simulink model "Rudder_system_control2020_3"  (R2020a)
settings: Solver=VariableStepAuto  StartTime=0.0  StopTime=300  MaxStep=0.02  RelTol=1e-3  AbsTol=1e-3  EnableMultiTasking=on
undefined symbols (not defined in the file or in its folder): Fg, H, Js, sigbuilder_block
libraries: fl_lib x76, nesl_utility x15, sh_lib x2
CloseFcn:
  | try,close(h1_ssc_hydraulic_actuator_analog_control),end
  | clear h1_ssc_hydraulic_actuator_analog_control
  | 
  | clear simlog_ssc_hydraulic_actuator_analog_control
Description:
  | Hydraulic Actuator with Analog Position Controller
settings Model: Creator=MathWorks  LastModifiedBy=victo
settings SolverCC: AutoScaleAbsTol=off  AlgebraicLoopSolver=LineSearch
settings DataIOCC: LimitDataPoints=on  SaveFormat=Array  ReturnWorkspaceOutputs=off
settings OptimizationCC: LifeSpan=inf
settings DebuggingCC: SolverPrmCheckMsg=warning  AllowSymbolicDim=off  PregeneratedLibrarySubsystemCodeDiagnostic=none  SFUnexpectedBacktrackingDiag=warning  SFNoUnconditionalDefaultTransitionDiag=warning  SFExecutionAtInitializationDiag=none  ArithmeticOperatorsInVariantConditions=warning
settings HardwareCC: ProdBitPerPointer=32  ProdBitPerSizeT=32  ProdBitPerPtrDiffT=32  ProdLargestAtomicFloat=None  ProdIntDivRoundTo=Undefined  ProdEndianess=Unspecified  ProdWordSize=32  ProdHWDeviceType=32-bit Generic
settings ModelReferenceCC: PropagateSignalLabelsOutOfModel=off
settings SFSimCC: SimUseLocalCustomCode=off  CustomCodeUndefinedFunction=UseInterfaceOnly
settings RTWCC: RTWUseLocalCustomCode=off
settings CodeAppCC: StateflowObjectComments=on
settings GRTTargetCC: TargetLangStandard=C89/C90 (ANSI)
settings ConfigComp: CovMetricSettings=dw  CovHtmlReporting=on  CovSaveCumulativeToWorkspaceVar=on  CovSaveSingleToWorkspaceVar=on  CovExternalEMLEnable=off  CovSFcnEnable=off
settings SimscapeCC: SimscapeLogType=all  SimscapeLogSimulationStatistics=on  SimscapeLogName=simlog_ssc_hydraulic_actuator_analog_control  SimscapeLogDataHistory=10000

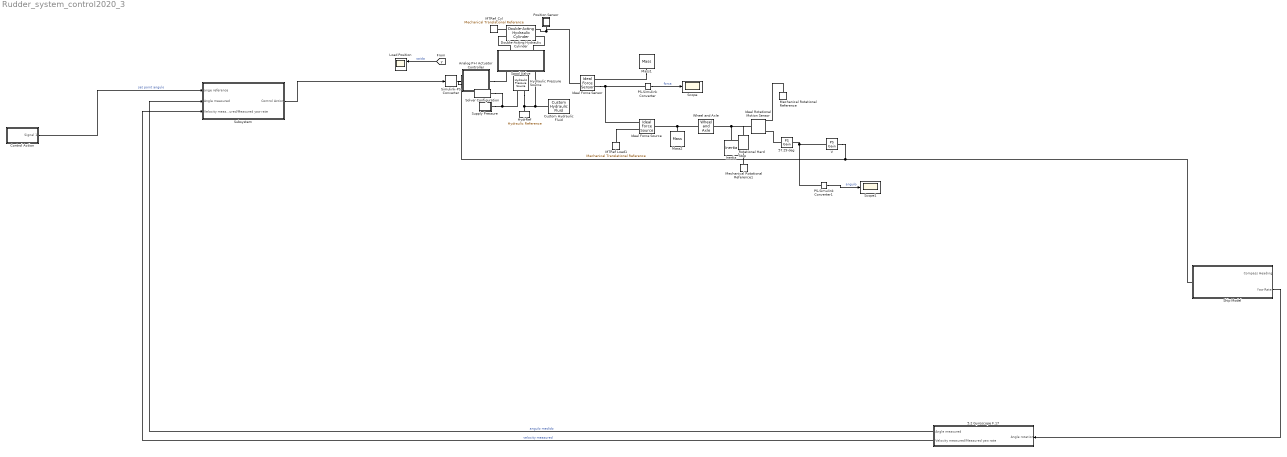
== system Rudder_system_control2020_3 ==
  5.2 Gyroscope F.17 : Subsystem
  57.29 deg : fl_lib/Physical Signals/Functions/PS Gain  gain=57.29 deg
      settings: SourceProductName=Foundation Library
  Analog P+I Actuator Controller : Subsystem
  Control Action : Subsystem  Tag=STV Subsys  LoadFcn=sigbuilder_block('load',[437.6 153 550.4 359.25 ]);  StartFcn=sigbuilder_block('start');  StopFcn=sigbuilder_block('stop');  ClipboardFcn=sigbuilder_block('clipboard');  mask(Sigbuilder block){tuvar=[0:10]}
      mask help: Simulink:masks:SigbuilderBlock_MD
      mask init:
      | if ~strcmp(get_param(bdroot(gcbh),'SimulationStatus'),'stopped') tuvar = sigbuilder_block('maskInit'); end
      settings: CopyFcn=sigbuilder_block('copy');  DeleteFcn=sigbuilder_block('delete');  ModelCloseFcn=sigbuilder_block('modelClose');  PreSaveFcn=sigbuilder_block('preSave');  PauseFcn=sigbuilder_block('pause');  ContinueFcn=sigbuilder_block('continue');  NameChangeFcn=sigbuilder_block('namechange');  OpenFcn=sigbuilder_block('open',[437.6 153 550.4 359.25 ]);  CloseFcn=sigbuilder_block('close');
      mask Display: plot(0, 0, 100, 100,[2, 2, 32, 32, 2], [68, 8, 8, 68, 68],[32, 2], [38, 38], [32, 19, 2],[53, 60, 44], [32, 17, 17, 2],[16, 16, 31, 31]);txt = getActiveGroup(gcbh);text(2, 100, txt,'verticalAlignment', 'top');
  Custom Hydraulic Fluid : fl_lib/Hydraulic/Hydraulic Utilities/Custom Hydraulic Fluid  density=850 kg/m^3  viscosity_kin=1.8e-05 m^2/s  bulk=8e+08 Pa  alpha=0.005  range_error=2
      settings: SourceProductName=Foundation Library  InternalSimscapePortConfiguration="{\"Bottom\":[],\"Left\":[],\"Right\":[{\"id\":\"G\",\"label\":\"\",\"type\":\"foundation.hydraulic.hydraulic\"}],\"Top\":[]}"
  Double-Acting Hydraulic Cylinder : sh_lib/Hydraulic Cylinders/Double-Acting Hydraulic Cylinder  area_A=PistonArea m^2  area_B=PistonArea m^2  stroke=PistonStroke m  init_pos=0 m  dead_vol_A=1e-4 m^3  dead_vol_B=1e-4 m^3  init_pressure_A=0 Pa  init_pressure_B=0 Pa  k_sh=1.4  stiff=1e6 N/m  D=150 N/(m/s)  hardstop_model=1  transition=0.1 mm  or=1
      settings: SourceProductBaseCode=SH  InternalSimscapePortConfiguration="{\"Bottom\":[],\"Left\":[{\"id\":\"C\",\"label\":\"C\",\"type\":\"foundation.mechanical.translational.translational\"},{\"id\":\"A\",\"label\":\"A\",\"type\":\"foundation.hydraulic.hydraulic\"}],\"Right\":[{\"id\":\"R\",\"label\":\"R\",\"type\":\"foundation.mechanical.translational.translational\"},{\"id\":\"B\",\"label\":\"B\",\"type\":\"foundation.hydraulic.hydraulic\"}],\"Top\":[]}"
  HydrRef : fl_lib/Hydraulic/Hydraulic Elements/Hydraulic Reference
      settings: SourceProductName=Foundation Library
  Hydraulic Pressure Source : fl_lib/Hydraulic/Hydraulic Sources/Hydraulic Pressure Source
      settings: SourceProductName=Foundation Library  InternalSimscapePortConfiguration="{\"Bottom\":[],\"Left\":[{\"id\":\"P\",\"label\":\"P\",\"type\":\"foundation.hydraulic.hydraulic\"}],\"Right\":[{\"id\":\"S\",\"label\":\"S\",\"type\":\"input\"},{\"id\":\"T\",\"label\":\"T\",\"type\":\"foundation.hydraulic.hydraulic\"}],\"Top\":[]}"
  Ideal Force Sensor : fl_lib/Mechanical/Mechanical Sensors/Ideal Force Sensor
  Ideal Force Source : fl_lib/Mechanical/Mechanical Sources/Ideal Force Source
  Ideal Rotational Motion Sensor : fl_lib/Mechanical/Mechanical Sensors/Ideal Rotational Motion Sensor  wrap_angle=simscape.enum.onoff.off  offset=0 rad
  Inertia : fl_lib/Mechanical/Rotational Elements/Inertia  inertia=Izz kg*m^2  w_specify=off  w_priority=High  w=0 rad/s  w_nominal_specify=off  w_nominal_unit=rad/s  w_nominal_value=1  t_specify=off  t_priority=None  t=0 N*m  t_nominal_specify=off  t_nominal_unit=N*m  t_nominal_value=1
  Load Position : Scope  NumInputPorts=2
  MTRef Load1 : fl_lib/Mechanical/Translational Elements/Mechanical Translational Reference
      settings: SourceProductName=Foundation Library
  MTRef_Cyl : fl_lib/Mechanical/Translational Elements/Mechanical Translational Reference
      settings: SourceProductName=Foundation Library
  Mass1 : fl_lib/Mechanical/Translational Elements/Mass  mass=PistonMass kg  v_specify=off  v_priority=High  v=0 m/s  v_nominal_specify=off  v_nominal_unit=m/s  v_nominal_value=1  f_specify=off  f_priority=High  f=0 N  f_nominal_specify=off  f_nominal_unit=N  f_nominal_value=1
      settings: SourceProductName=Foundation Library
  Mass2 : fl_lib/Mechanical/Translational Elements/Mass  mass=mrudder kg  v_specify=off  v_priority=High  v=0 m/s  v_nominal_specify=off  v_nominal_unit=m/s  v_nominal_value=1  f_specify=off  f_priority=High  f=0 N  f_nominal_specify=off  f_nominal_unit=N  f_nominal_value=1
      settings: SourceProductName=Foundation Library
  Mechanical Rotational Reference : fl_lib/Mechanical/Rotational Elements/Mechanical Rotational Reference
  Mechanical Rotational Reference1 : fl_lib/Mechanical/Rotational Elements/Mechanical Rotational Reference
  PS-Simulink Converter : nesl_utility/PS-Simulink Converter  PhysicalDomain=network_engine_domain  SubClassName=ps_output  LeftPortType=input  RightPortType=output  PseudoPeriodic=off  Frequencies=[]  Unit=inherit  AffineConversion=off
  PS-Simulink Converter1 : nesl_utility/PS-Simulink Converter  PhysicalDomain=network_engine_domain  SubClassName=ps_output  LeftPortType=input  RightPortType=output  PseudoPeriodic=off  Frequencies=[]  Unit=inherit  AffineConversion=off
  Position Sensor : Subsystem
      mask Display: disp('y')
  Rotational Hard Stop : fl_lib/Mechanical/Rotational Elements/Rotational Hard Stop  upper_bnd=30 deg  lower_bnd=-30 deg  stiff_up=1e6 N*m/rad  stiff_low=1e6 N*m/rad  D_up=0.01 N*m/(rad/s)  D_low=0.01 N*m/(rad/s)  model=simscape.enum.hardstop.smooth  transition=0.001 rad  w_specify=off  w_priority=None  w=0 rad/s  w_nominal_specify=off  w_nominal_unit=rad/s  w_nominal_value=1  t_specify=off  t_priority=None  t=0 N*m  t_nominal_specify=off  t_nominal_unit=N*m  t_nominal_value=1  phi_specify=off  phi_priority=High  phi=0 rad  phi_nominal_specify=off  phi_nominal_unit=rad  phi_nominal_value=1
      settings: SourceProductBaseCode=SS
  Scope : Scope
  Scope1 : Scope
  Ship Model : Subsystem
  Simulink-PS Converter : nesl_utility/Simulink-PS Converter  PhysicalDomain=network_engine_domain  SubClassName=ps_input  LeftPortType=input  RightPortType=output  PseudoPeriodic=off  Frequencies=[]  NoiseDistribution=none  NoiseParameters=[]  Unit=V  AffineConversion=off  FilteringAndDerivatives=zero  SimscapeFilterOrder=1  InputFilterTimeConstant=.001  UdotUserProvided=0
      settings: SourceProductName=Utilities
  Solver Configuration : nesl_utility/Solver Configuration  PhysicalDomain=network_engine_domain  SubClassName=solver  LeftPortType=input  RightPortType=generic  Tones=[]  Harmonics=[]  SimulateNoise=off  Profile=off  UseLocalSampling=off  EnableSwitchedLinearOptims=on  FrequencyDomain=off  UseCCode=off  RelTol=0.001  AbsTol=1e-06  MinStep=1e-09  ToWorkspace=off  RevertToSquareIcSolve=off  NumHomotopyIterations=100  PhasorMode=off  PhasorModeNumHarmonics=1  DoDC=off  ResidualTolerance=1e-9  UseLocalSolver=off  LocalSolverChoice=NE_BACKWARD_EULER_ADVANCER  LocalSolverSampleTime=0.001  DoFixedCost=off  MaxNonlinIter=3  MaxModeIter=2  LinearAlgebra=auto  EquationFormulation=NE_TIME_EF  DelaysMemoryBudget=1024  AutomaticFiltering=on  FilteringTimeConstant=0.001  PartitionStorageMethod=AS_NEEDED  PartitionMemoryBudget=1024  PartitionMethod=ROBUST
      settings: SourceProductName=Utilities
  Spool Valve : Subsystem  Tag=PublishSubsystem  mask(Single-Stage Servo Valve){K_V=0.5, x_max=0.5, A_max=9, x_lap=0.02, A_leak=0.25, G=0.5e-3/(pi/2), J=1e-4, lambda=0.01, R=10, L=2.5, Kt=0.04, R_controller=[10e3 10e3 10e3 100e3 50 100e3 10e3]}
      mask prompts: K_V "Flow Coefficient:"; x_max "Spool displacement limit (mm)"; A_max "Maximum orifice area (mm^2)"; x_lap "Spool displacement range for leakage (mm)"; A_leak "Leakage area at x=0 (mm^2)"; G "Spool displacement per motor rotation (m/radian)"; J "Total inertia reflected to motor (kg m^2)"; lambda "Total damping reflected to motor (Nm/(rad/s))"; R "Torque motor winding resistance (ohms)"; L "Torque motor winding inductance (H)"; Kt "Torque motor torque constant (Nm/A)"; R_controller "Motor controller resistance values [R1 R2 R3 R4 R5 R6 R7] (ohms)"
      mask help: Models a spool valve actuated directly by a torque motor.
      mask Display:
      | % Plot icon
      | plot([0;337.311462499201;337.311462499201;0;0], [566.910021007061;566.910021007061;0;0;566.910021007061])
      | plot([84.6585631370544;241.503668949008], [353;353])
      | plot([84.6585631370544;241.503668949008], [214;214])
      | plot([84.6585631370544;241.503668949008;241.503668949008;84.6585631370544;84.6585631370544], [491;491;76;76;491])
      | plot([84.6585631370544;241.503668949008], [449;449])
      | plot([241.503668949008;210.071657784283], [310;310])
      | plot([210.071657784283;210.071657784283;210.071657784283], [326;295;310.414731502533])
      | plot([241.503668949008;210.071657784283], [257;257])
      | plot([210.071657784283;210.071657784283;210.071657784283], [272;241;236.464468762279])
      | plot([84.6585631370544;115.964594297111], [257;257])
      | plot([115.964594297111;115.964594297111;115.964594297111], [272;241;236.464468762279])
      | plot([84.6585631370544;115.964594297111], [310;310])
      | plot([115.964594297111;115.964594297111;115.964594297111], [326;295;310.414731502533])
      | plot([84.6585631370544;241.503668949008], [185;110])
      | plot([241.503668949008;84.6585631370544], [185;110])
      | plot([84.6585631370544;241.503668949008], [395;395])
      | patch([85.0365031510592;110.547454096377;121.885654516518;85.0365031510592], [110;140;120;110], [0;0;0])
      | plot([85.0365031510592;110.547454096377;121.885654516518;85.0365031510592], [110;140;120;110])
      | patch([240.936758928001;204.087607562542;215.425807982683;240.936758928001], [109;120;140;109], [0;0;0])
      | 
      | plot([240.936758928001;204.087607562542;215.425807982683;240.936758928001], [109;120;140;109])
      | patch([83.6507230997086;127.554754726589;127.554754726589;83.6507230997086], [394;405;384;394], [0;0;0])
      | plot([83.6507230997086;127.554754726589;127.554754726589;83.6507230997086], [394;405;384;394])
      | patch([245.283069089055;201.253057457507;201.253057457507;245.283069089055], [451;461;440;451], [0;0;0])
      | plot([245.283069089055;201.253057457507;201.253057457507;245.283069089055], [451;461;440;451])
      | 
      | % Port labels
      | color('red')
      | port_label('LConn', 1,'S')
      | port_label('LConn', 2,'P')
      | port_label('LConn', 3,'T')
      | port_label('RConn', 1,'A')
      | port_label('RConn', 2,'B')
      | color('black')
  Subsystem : Subsystem
  Supply Pressure : Subsystem
  V : fl_lib/Physical Signals/Functions/PS Gain  gain=1 V
      settings: SourceProductName=Foundation Library
  Wheel and Axle : fl_lib/Mechanical/Mechanisms/Wheel and Axle  R=0.05 m  or=1  t_specify=off  t_priority=None  t=0 N*m  t_nominal_specify=off  t_nominal_unit=N*m  t_nominal_value=1  f_specify=off  f_priority=None  f=0 N  f_nominal_specify=off  f_nominal_unit=N  f_nominal_value=1
  wires:
  [y] -> Load Position/1  "saida"
  PS-Simulink Converter/1 -> Scope/1  "forca"
  PS-Simulink Converter1/1 -> Scope1/1  "angulo"
  Subsystem/1(Control Action) -> Simulink-PS Converter/1
  5.2 Gyroscope F.17/1(Angle measured) -> Subsystem/2(Angle measured)  "angulo medido"
  5.2 Gyroscope F.17/2(Velocity measured/Measured yaw rate) -> Subsystem/3(Velocity measured/Measured yaw rate)  "velocity measured"
  Control Action/1(Signal 1) -> Subsystem/1(ange reference)  "set point angulo"
  Ship Model/2(Yaw Rate) -> 5.2 Gyroscope F.17/1(Angle rotation)
  connections:
  Custom Hydraulic Fluid/RConn1 -- Hydraulic Pressure Source/RConn2 -- HydrRef/LConn1 -- Spool Valve/LConn3
  Spool Valve/RConn2 -- Double-Acting Hydraulic Cylinder/RConn2
  Spool Valve/RConn1 -- Double-Acting Hydraulic Cylinder/LConn2
  Simulink-PS Converter/RConn1 -- Analog P+I Actuator Controller/LConn2
  Hydraulic Pressure Source/LConn1 -- Spool Valve/LConn2
  Position Sensor/RConn1 -- Ideal Force Sensor/LConn1 -- Double-Acting Hydraulic Cylinder/RConn1
  Supply Pressure/RConn1 -- Solver Configuration/RConn1 -- Hydraulic Pressure Source/RConn1
  Double-Acting Hydraulic Cylinder/LConn1 -- MTRef_Cyl/LConn1
  Ideal Force Sensor/RConn2 -- Ideal Force Source/RConn1 -- PS-Simulink Converter/LConn1
  Mass1/LConn1 -- Ideal Force Sensor/RConn1
  MTRef Load1/LConn1 -- Ideal Force Source/RConn2
  Mass2/LConn1 -- Wheel and Axle/RConn1 -- Ideal Force Source/LConn1
  Inertia/LConn1 -- Rotational Hard Stop/LConn1 -- Ideal Rotational Motion Sensor/LConn1 -- Wheel and Axle/LConn1
  Mechanical Rotational Reference/LConn1 -- Ideal Rotational Motion Sensor/RConn1
  57.29 deg/LConn1 -- Ideal Rotational Motion Sensor/RConn3
  PS-Simulink Converter1/LConn1 -- V/LConn1 -- 57.29 deg/RConn1
  Mechanical Rotational Reference1/LConn1 -- Rotational Hard Stop/RConn1
  V/RConn1 -- Ship Model/LConn1 -- Analog P+I Actuator Controller/LConn1
  Analog P+I Actuator Controller/RConn1 -- Spool Valve/LConn1

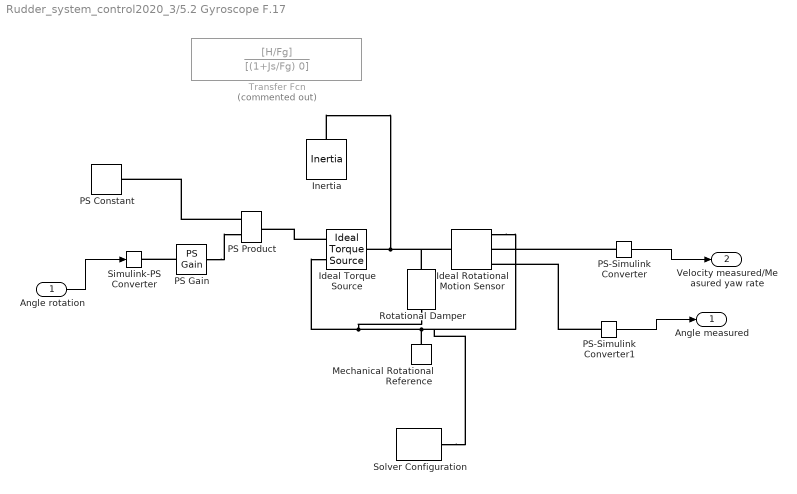
== system Rudder_system_control2020_3/5.2 Gyroscope F.17 ==
  Angle rotation : Inport
  Ideal Rotational Motion Sensor : fl_lib/Mechanical/Mechanical Sensors/Ideal Rotational Motion Sensor  wrap_angle=simscape.enum.onoff.off  offset=0 rad
  Ideal Torque Source : fl_lib/Mechanical/Mechanical Sources/Ideal Torque Source
  Inertia : fl_lib/Mechanical/Rotational Elements/Inertia  inertia=0.08 kg*m^2  w_specify=off  w_priority=High  w=0 rad/s  w_nominal_specify=off  w_nominal_unit=rad/s  w_nominal_value=1  t_specify=off  t_priority=None  t=0 N*m  t_nominal_specify=off  t_nominal_unit=N*m  t_nominal_value=1
  Mechanical Rotational Reference : fl_lib/Mechanical/Rotational Elements/Mechanical Rotational Reference
  PS Constant : fl_lib/Physical Signals/Sources/PS Constant  constant=1
  PS Gain : fl_lib/Physical Signals/Functions/PS Gain  gain=0.017
  PS Product : fl_lib/Physical Signals/Functions/PS Product
  PS-Simulink Converter : nesl_utility/PS-Simulink Converter  PhysicalDomain=network_engine_domain  SubClassName=ps_output  LeftPortType=input  RightPortType=output  PseudoPeriodic=off  Frequencies=[]  Unit=inherit  AffineConversion=off
  PS-Simulink Converter1 : nesl_utility/PS-Simulink Converter  PhysicalDomain=network_engine_domain  SubClassName=ps_output  LeftPortType=input  RightPortType=output  PseudoPeriodic=off  Frequencies=[]  Unit=inherit  AffineConversion=off
  Rotational Damper : fl_lib/Mechanical/Rotational Elements/Rotational Damper  D=1 N*m/(rad/s)  w_specify=off  w_priority=None  w=0 rad/s  w_nominal_specify=off  w_nominal_unit=rad/s  w_nominal_value=1  t_specify=off  t_priority=None  t=0 N*m  t_nominal_specify=off  t_nominal_unit=N*m  t_nominal_value=1
  Simulink-PS Converter : nesl_utility/Simulink-PS Converter  PhysicalDomain=network_engine_domain  SubClassName=ps_input  LeftPortType=input  RightPortType=output  PseudoPeriodic=off  Frequencies=[]  NoiseDistribution=none  NoiseParameters=[]  Unit=1  AffineConversion=off  FilteringAndDerivatives=provide  SimscapeFilterOrder=1  InputFilterTimeConstant=0.001  UdotUserProvided=0
  Solver Configuration : nesl_utility/Solver Configuration  PhysicalDomain=network_engine_domain  SubClassName=solver  LeftPortType=input  RightPortType=generic  Tones=[]  Harmonics=[]  SimulateNoise=off  Profile=off  UseLocalSampling=off  EnableSwitchedLinearOptims=on  FrequencyDomain=off  UseCCode=off  RelTol=0.001  AbsTol=1e-06  MinStep=1e-09  ToWorkspace=off  RevertToSquareIcSolve=off  NumHomotopyIterations=100  PhasorMode=off  PhasorModeNumHarmonics=1  DoDC=off  ResidualTolerance=1e-09  UseLocalSolver=off  LocalSolverChoice=NE_BACKWARD_EULER_ADVANCER  LocalSolverSampleTime=0.001  DoFixedCost=off  MaxNonlinIter=3  MaxModeIter=2  LinearAlgebra=auto  EquationFormulation=NE_TIME_EF  DelaysMemoryBudget=1024  AutomaticFiltering=on  FilteringTimeConstant=0.001  PartitionStorageMethod=AS_NEEDED  PartitionMemoryBudget=1024  PartitionMethod=ROBUST
  Transfer Fcn : TransferFcn  Commented=on  Numerator=[H/Fg]  Denominator=[(1+Js/Fg) 0]
  Angle measured : Outport
  Velocity measured/Measured yaw rate : Outport  Port=2
  wires:
  Angle rotation/1 -> Simulink-PS Converter/1
  PS-Simulink Converter/1 -> Velocity measured/Measured yaw rate/1
  PS-Simulink Converter1/1 -> Angle measured/1
  connections:
  PS Product/LConn1 -- PS Constant/RConn1
  PS Gain/LConn1 -- Simulink-PS Converter/RConn1
  PS Gain/RConn1 -- PS Product/LConn2
  Ideal Torque Source/RConn1 -- PS Product/RConn1
  Mechanical Rotational Reference/LConn1 -- Solver Configuration/RConn1 -- Ideal Rotational Motion Sensor/RConn1 -- Rotational Damper/RConn1 -- Ideal Torque Source/RConn2
  Inertia/LConn1 -- Rotational Damper/LConn1 -- Ideal Rotational Motion Sensor/LConn1 -- Ideal Torque Source/LConn1
  PS-Simulink Converter/LConn1 -- Ideal Rotational Motion Sensor/RConn2
  PS-Simulink Converter1/LConn1 -- Ideal Rotational Motion Sensor/RConn3

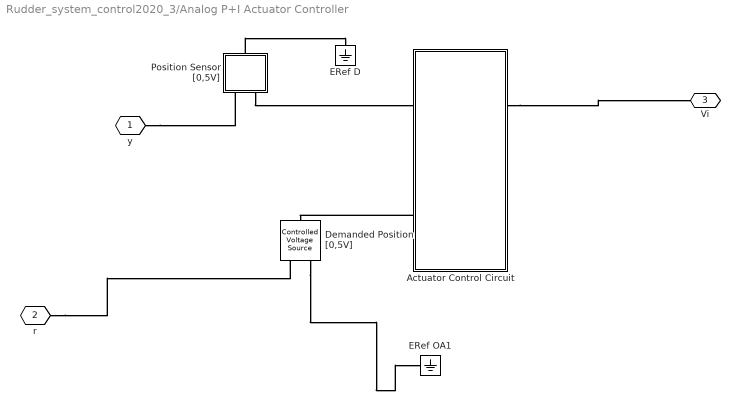
== system Rudder_system_control2020_3/Analog P+I Actuator Controller ==
  Actuator Control Circuit : Subsystem  Tag=PublishSubsystem
  Demanded Position [0,5V] : fl_lib/Electrical/Electrical Sources/Controlled Voltage Source
      settings: SourceProductName=Foundation Library
  ERef D : fl_lib/Electrical/Electrical Elements/Electrical Reference
      settings: SourceProductName=Foundation Library
  ERef OA1 : fl_lib/Electrical/Electrical Elements/Electrical Reference
      settings: SourceProductName=Foundation Library
  Position Sensor [0,5V] : Subsystem
  y : PMIOPort  Tag=PMCPort  Side=Left
  r : PMIOPort  Tag=PMCPort  Port=2  Side=Left
  Vi : PMIOPort  Port=3  Side=Right
  connections:
  y/RConn1 -- Position Sensor [0,5V]/LConn1
  r/RConn1 -- Demanded Position [0,5V]/RConn1
  Actuator Control Circuit/LConn2 -- Demanded Position [0,5V]/LConn1
  Position Sensor [0,5V]/RConn1 -- ERef D/LConn1
  Position Sensor [0,5V]/LConn2 -- Actuator Control Circuit/LConn1
  Actuator Control Circuit/RConn1 -- Vi/RConn1
  Demanded Position [0,5V]/RConn2 -- ERef OA1/LConn1

== system Rudder_system_control2020_3/Control Action ==
  Demux : Demux  Tag=STV Demux  Outputs=1
      settings: DisplayOption=none
  FromWs : FromWorkspace  Tag=STV FromWs  VariableName=tuvar
      SigBuilderData=|
      | common.afterFinalStr = 'Extrapolate'
      | common.sampleTime = 0
      | dataSet.timeRange = [0 10]
      | dataSet.name = 'Group 1'
      | sbobj.Groups.Name = 'Group 1'
      | sbobj.Groups.Signals.Name = 'Signal 1'
      | sbobj.Groups.Signals.XData = [0 1.02 1.02 10]
      | sbobj.Groups.Signals.YData = [0 0 1 1]
  Signal 1 : Outport  Tag=STV Outport
  wires:
  Demux/1 -> Signal 1/1
  FromWs/1 -> Demux/1

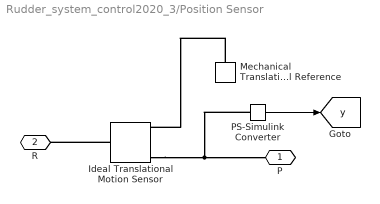
== system Rudder_system_control2020_3/Position Sensor ==
  Ideal Translational Motion Sensor : fl_lib/Mechanical/Mechanical Sensors/Ideal Translational Motion Sensor  offset=0 m
  Mechanical Translational Reference : fl_lib/Mechanical/Translational Elements/Mechanical Translational Reference
  PS-Simulink Converter : nesl_utility/PS-Simulink Converter  PhysicalDomain=network_engine_domain  SubClassName=ps_output  LeftPortType=input  RightPortType=output  PseudoPeriodic=off  Frequencies=[]  Unit=inherit  AffineConversion=off
  P : PMIOPort  Side=Left
  R : PMIOPort  Port=2  Side=Right
  tag scope: y=global
  wires:
  PS-Simulink Converter/1 -> [y]
  connections:
  Ideal Translational Motion Sensor/LConn1 -- R/RConn1
  Ideal Translational Motion Sensor/RConn3 -- PS-Simulink Converter/LConn1 -- P/RConn1
  Mechanical Translational Reference/LConn1 -- Ideal Translational Motion Sensor/RConn1

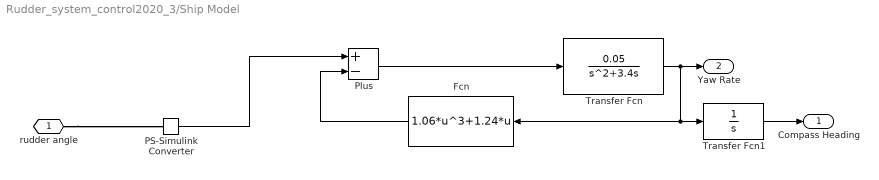
== system Rudder_system_control2020_3/Ship Model ==
  Fcn : Fcn  Expr=1.06*u^3+1.24*u
  PS-Simulink Converter : nesl_utility/PS-Simulink Converter  PhysicalDomain=network_engine_domain  SubClassName=ps_output  LeftPortType=input  RightPortType=output  PseudoPeriodic=off  Frequencies=[]  Unit=inherit  AffineConversion=off
  Plus : Sum  Inputs=+-
  Transfer Fcn : TransferFcn  Numerator=[0.05]  Denominator=[1 3.4 0]
  Transfer Fcn1 : TransferFcn  Denominator=[1 0]
  rudder angle : PMIOPort  Side=Left
  Compass Heading : Outport
  Yaw Rate : Outport  Port=2
  wires:
  Transfer Fcn1/1 -> Compass Heading/1
  Fcn/1 -> Plus/2
  Transfer Fcn/1 -> Fcn/1, Transfer Fcn1/1, Yaw Rate/1
  Plus/1 -> Transfer Fcn/1
  PS-Simulink Converter/1 -> Plus/1
  connections:
  rudder angle/RConn1 -- PS-Simulink Converter/LConn1

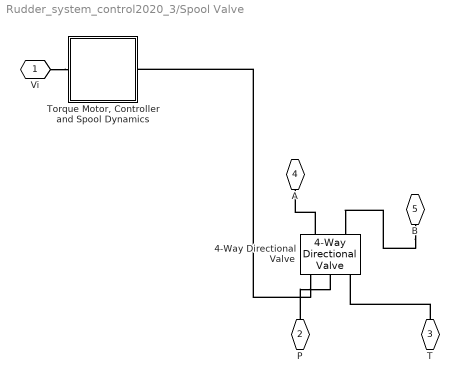
== system Rudder_system_control2020_3/Spool Valve ==
  4-Way Directional Valve : sh_lib/Valves/Directional Valves/4-Way Directional Valve  area_spec=sh.valves.directional_valves.enum.area_spec.identical  x_0_P_A=0 m  x_0_P_B=0 m  x_0_A_T=0 m  x_0_B_T=0 m  mdl_type_identical=sh.valves.directional_valves.enum.mdl_type.linear  mdl_type_different=sh.valves.directional_valves.enum.mdl_type.linear  opening_max=0.005 m  area_max=0.5e-4 m^2  opening_max_P_A=0.005 m  area_max_P_A=0.5e-4 m^2  opening_max_P_B=0.005 m  area_max_P_B=0.5e-4 m^2  opening_max_A_T=0.005 m  area_max_A_T=0.5e-4 m^2  opening_max_B_T=0.005 m  area_max_B_T=0.5e-4 m^2  opening_area_tab=[-.002, 0, .002, .005, .015] m  area_tab=[1e-09, 2.0352e-07, 4.0736e-05, .00011438, .00034356] m^2  opening_flow_rate_tab=[-.002, 0, .002, .005, .015] m  pressure_tab=[-10000000, -5000000, -2000000, 2000000, 5000000, 10000000] Pa  flow_rate_tab=[-1e-07, -7.0711e-08, -4.4721e-08, 4.4721e-08, 7.0711e-08, 1e-07; -2.0352e-05, -1.4391e-05, -9.1017e-06, 9.1017e-06, 1.4391e-05, 2.0352e-05; -.0040736, -.0028805, -.0018218, .0018218, .0028805, .0040736; -.011438, -.0080879, -.0051152, .0051152, .0080879, .011438; -.034356, -.024293, -.015364, .015364, .024293, .034356] m^3/s  opening_area_tab_P_A=[-.002, 0, .002, .005, .015] m  area_tab_P_A=[1e-09, 2.0352e-07, 4.0736e-05, .00011438, .00034356] m^2  opening_flow_rate_tab_P_A=[-.002, 0, .002, .005, .015] m  pressure_tab_P_A=[-10000000, -5000000, -2000000, 2000000, 5000000, 10000000] Pa  flow_rate_tab_P_A=[-1e-07, -7.0711e-08, -4.4721e-08, 4.4721e-08, 7.0711e-08, 1e-07; -2.0352e-05, -1.4391e-05, -9.1017e-06, 9.1017e-06, 1.4391e-05, 2.0352e-05; -.0040736, -.0028805, -.0018218, .0018218, .0028805, .0040736; -.011438, -.0080879, -.0051152, .0051152, .0080879, .011438; -.034356, -.024293, -.015364, .015364, .024293, .034356] m^3/s  opening_area_tab_P_B=[-.002, 0, .002, .005, .015] m  area_tab_P_B=[1e-09, 2.0352e-07, 4.0736e-05, .00011438, .00034356] m^2  opening_flow_rate_tab_P_B=[-.002, 0, .002, .005, .015] m  pressure_tab_P_B=[-10000000, -5000000, -2000000, 2000000, 5000000, 10000000] Pa  flow_rate_tab_P_B=[-1e-07, -7.0711e-08, -4.4721e-08, 4.4721e-08, 7.0711e-08, 1e-07; -2.0352e-05, -1.4391e-05, -9.1017e-06, 9.1017e-06, 1.4391e-05, 2.0352e-05; -.0040736, -.0028805, -.0018218, .0018218, .0028805, .0040736; -.011438, -.0080879, -.0051152, .0051152, .0080879, .011438; -.034356, -.024293, -.015364, .015364, .024293, .034356] m^3/s  opening_area_tab_A_T=[-.002, 0, .002, .005, .015] m  area_tab_A_T=[1e-09, 2.0352e-07, 4.0736e-05, .00011438, .00034356] m^2  opening_flow_rate_tab_A_T=[-.002, 0, .002, .005, .015] m  pressure_tab_A_T=[-10000000, -5000000, -2000000, 2000000, 5000000, 10000000] Pa  flow_rate_tab_A_T=[-1e-07, -7.0711e-08, -4.4721e-08, 4.4721e-08, 7.0711e-08, 1e-07; -2.0352e-05, -1.4391e-05, -9.1017e-06, 9.1017e-06, 1.4391e-05, 2.0352e-05; -.0040736, -.0028805, -.0018218, .0018218, .0028805, .0040736; -.011438, -.0080879, -.0051152, .0051152, .0080879, .011438; -.034356, -.024293, -.015364, .015364, .024293, .034356] m^3/s  opening_area_tab_B_T=[-.002, 0, .002, .005, .015] m  area_tab_B_T=[1e-09, 2.0352e-07, 4.0736e-05, .00011438, .00034356] m^2  opening_flow_rate_tab_B_T=[-.002, 0, .002, .005, .015] m  pressure_tab_B_T=[-10000000, -5000000, -2000000, 2000000, 5000000, 10000000] Pa  flow_rate_tab_B_T=[-1e-07, -7.0711e-08, -4.4721e-08, 4.4721e-08, 7.0711e-08, 1e-07; -2.0352e-05, -1.4391e-05, -9.1017e-06, 9.1017e-06, 1.4391e-05, 2.0352e-05; -.0040736, -.0028805, -.0018218, .0018218, .0028805, .0040736; -.011438, -.0080879, -.0051152, .0051152, .0080879, .011438; -.034356, -.024293, -.015364, .015364, .024293, .034356] m^3/s  interp_method_identical=sh.valves.directional_valves.enum.interp_method.linear  interp_method_different=sh.valves.directional_valves.enum.interp_method.linear  extrap_method_identical=sh.valves.directional_valves.enum.extrap_method.linear  extrap_method_different=sh.valves.directional_valves.enum.extrap_method.linear  A_leak=1e-12 m^2  C_d=0.7  lam_spec=sh.valves.directional_valves.enum.lam_spec.pressure_ratio  B_lam=0.999  Re_cr=12
      settings: SourceProductBaseCode=SH  InternalSimscapePortConfiguration="{\"Bottom\":[],\"Left\":[{\"id\":\"A\",\"label\":\"A\",\"type\":\"foundation.hydraulic.hydraulic\"},{\"id\":\"B\",\"label\":\"B\",\"type\":\"foundation.hydraulic.hydraulic\"}],\"Right\":[{\"id\":\"S\",\"label\":\"S\",\"type\":\"input\"},{\"id\":\"P\",\"label\":\"P\",\"type\":\"foundation.hydraulic.hydraulic\"},{\"id\":\"T\",\"label\":\"T\",\"type\":\"foundation.hydraulic.hydraulic\"}],\"Top\":[]}"
  "Torque Motor, Controller and Spool Dynamics" : Subsystem
  Vi : PMIOPort  Tag=PMCPort  Side=Left
  P : PMIOPort  Tag=PMCPort  Port=2  Side=Left
  T : PMIOPort  Tag=PMCPort  Port=3  Side=Left
  A : PMIOPort  Tag=PMCPort  Port=4  Side=Right
  B : PMIOPort  Tag=PMCPort  Port=5  Side=Right
  connections:
  Vi/RConn1 -- "Torque Motor, Controller and Spool Dynamics"/LConn1
  4-Way Directional Valve/RConn1 -- "Torque Motor, Controller and Spool Dynamics"/RConn1
  4-Way Directional Valve/LConn1 -- A/RConn1
  B/RConn1 -- 4-Way Directional Valve/LConn2
  P/RConn1 -- 4-Way Directional Valve/RConn2
  T/RConn1 -- 4-Way Directional Valve/RConn3

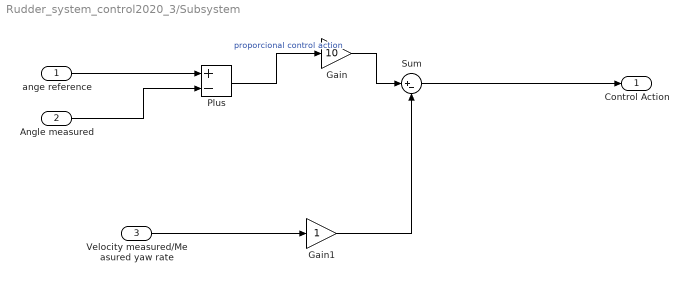
== system Rudder_system_control2020_3/Subsystem ==
  ange reference : Inport
  Angle measured : Inport  Port=2
  Velocity measured/Measured yaw rate : Inport  Port=3
  Gain : Gain  Gain=10
  Gain1 : Gain
  Plus : Sum  Inputs=+-
  Sum : Sum  Inputs=|+-
  Control Action : Outport
  wires:
  Sum/1 -> Control Action/1
  Plus/1 -> Gain/1  "proporcional control action"
  ange reference/1 -> Plus/1
  Angle measured/1 -> Plus/2
  Gain/1 -> Sum/1
  Gain1/1 -> Sum/2
  Velocity measured/Measured yaw rate/1 -> Gain1/1

== system Rudder_system_control2020_3/Supply Pressure ==
  Supply Pressure : Constant  Value=200
  bar : nesl_utility/Simulink-PS Converter  PhysicalDomain=network_engine_domain  SubClassName=ps_input  LeftPortType=input  RightPortType=output  PseudoPeriodic=off  Frequencies=[]  NoiseDistribution=none  NoiseParameters=[]  Unit=bar  AffineConversion=off  FilteringAndDerivatives=zero  SimscapeFilterOrder=1  InputFilterTimeConstant=.001  UdotUserProvided=0
      settings: SourceProductName=Utilities
  S : PMIOPort  Side=Right
  wires:
  Supply Pressure/1 -> bar/1
  connections:
  bar/RConn1 -- S/RConn1

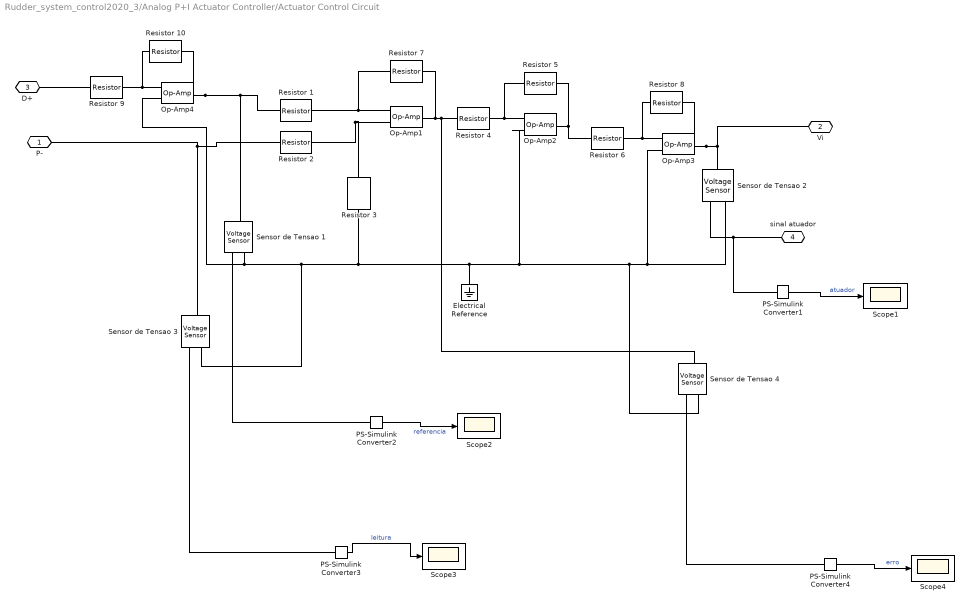
== system Rudder_system_control2020_3/Analog P+I Actuator Controller/Actuator Control Circuit ==
  Electrical Reference : fl_lib/Electrical/Electrical Elements/Electrical Reference
  Op-Amp{1..4} (4 alike) : fl_lib/Electrical/Electrical Elements/Op-Amp  outI_specify=off  outI_priority=None  outI=0 A  outI_nominal_specify=off  outI_nominal_unit=A  outI_nominal_value=1
  PS-Simulink Converter{1..4} (4 alike) : nesl_utility/PS-Simulink Converter  PhysicalDomain=network_engine_domain  SubClassName=ps_output  LeftPortType=input  RightPortType=output  PseudoPeriodic=off  Frequencies=[]  Unit=inherit  AffineConversion=off
  Resistor {1..10} (10 alike) : fl_lib/Electrical/Electrical Elements/Resistor  R=1 Ohm  i_specify=off  i_priority=None  i=0 A  i_nominal_specify=off  i_nominal_unit=A  i_nominal_value=1  v_specify=off  v_priority=None  v=0 V  v_nominal_specify=off  v_nominal_unit=V  v_nominal_value=1
  Scope{1..4} (4 alike) : Scope
  Sensor de Tensao {1..4} (4 alike) : fl_lib/Electrical/Electrical Sensors/Voltage Sensor
  P- : PMIOPort  Side=Left
  Vi : PMIOPort  Port=2  Side=Right
  D+ : PMIOPort  Port=3  Side=Left
  sinal atuador : PMIOPort  Port=4  Side=Right
  wires:
  PS-Simulink Converter1/1 -> Scope1/1  "atuador"
  PS-Simulink Converter2/1 -> Scope2/1  "referencia"
  PS-Simulink Converter3/1 -> Scope3/1  "leitura"
  PS-Simulink Converter4/1 -> Scope4/1  "erro"
  connections:
  D+/RConn1 -- Resistor 9/LConn1
  Resistor 9/RConn1 -- Resistor 10/LConn1 -- Op-Amp4/LConn2
  Resistor 5/RConn1 -- Op-Amp2/RConn1 -- Resistor 6/LConn1
  Resistor 6/RConn1 -- Resistor 8/LConn1 -- Op-Amp3/LConn2
  Op-Amp1/RConn1 -- Resistor 7/RConn1 -- Resistor 4/LConn1 -- Sensor de Tensao 4/LConn1
  Op-Amp3/RConn1 -- Resistor 8/RConn1 -- Vi/RConn1 -- Sensor de Tensao 2/LConn1
  Resistor 2/RConn1 -- Op-Amp1/LConn1 -- Resistor 3/LConn1
  Op-Amp4/LConn1 -- Sensor de Tensao 1/RConn2 -- Sensor de Tensao 3/RConn2 -- Resistor 3/RConn1 -- Electrical Reference/LConn1 -- Op-Amp2/LConn1 -- Sensor de Tensao 4/RConn2 -- Sensor de Tensao 2/RConn2 -- Op-Amp3/LConn1
  Resistor 5/LConn1 -- Op-Amp2/LConn2 -- Resistor 4/RConn1
  Op-Amp1/LConn2 -- Resistor 7/LConn1 -- Resistor 1/RConn1
  sinal atuador/RConn1 -- Sensor de Tensao 2/RConn1 -- PS-Simulink Converter1/LConn1
  Op-Amp4/RConn1 -- Resistor 10/RConn1 -- Sensor de Tensao 1/LConn1 -- Resistor 1/LConn1
  Resistor 2/LConn1 -- Sensor de Tensao 3/LConn1 -- P-/RConn1
  Sensor de Tensao 1/RConn1 -- PS-Simulink Converter2/LConn1
  Sensor de Tensao 3/RConn1 -- PS-Simulink Converter3/LConn1
  Sensor de Tensao 4/RConn1 -- PS-Simulink Converter4/LConn1

== system Rudder_system_control2020_3/Analog P+I Actuator Controller/Position Sensor [0,5V] ==
  Controlled Voltage Source : fl_lib/Electrical/Electrical Sources/Controlled Voltage Source
      settings: SourceProductName=Foundation Library
  + : PMIOPort  Side=Right
  y : PMIOPort  Port=2  Side=Left
  - : PMIOPort  Port=3  Side=Left
  connections:
  +/RConn1 -- Controlled Voltage Source/LConn1
  -/RConn1 -- Controlled Voltage Source/RConn2
  Controlled Voltage Source/RConn1 -- y/RConn1

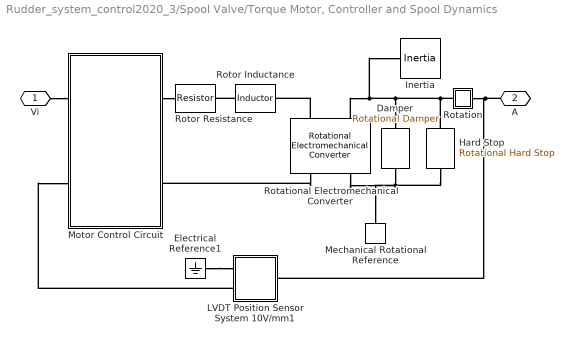
== system Rudder_system_control2020_3/Spool Valve/Torque Motor, Controller and Spool Dynamics ==
  Damper : fl_lib/Mechanical/Rotational Elements/Rotational Damper  D=lambda N*m/(rad/s)  w_specify=off  w_priority=High  w=0 rad/s  w_nominal_specify=off  w_nominal_unit=rad/s  w_nominal_value=1  t_specify=off  t_priority=High  t=0 N*m  t_nominal_specify=off  t_nominal_unit=N*m  t_nominal_value=1
      settings: SourceProductName=Foundation Library
  Electrical Reference1 : fl_lib/Electrical/Electrical Elements/Electrical Reference
      settings: SourceProductName=Foundation Library
  Hard Stop : fl_lib/Mechanical/Rotational Elements/Rotational Hard Stop  upper_bnd=x_max*1e-3/G rad  lower_bnd=-x_max*1e-3/G rad  stiff_up=1e+06 N*m/rad  stiff_low=1e+6 N*m/rad  D_up=0.05 N*m/(rad/s)  D_low=0.05 N*m/(rad/s)  model=3  transition=0.001 rad  w_specify=off  w_priority=High  w=0 rad/s  w_nominal_specify=off  w_nominal_unit=rad/s  w_nominal_value=1  t_specify=off  t_priority=High  t=0 N*m  t_nominal_specify=off  t_nominal_unit=N*m  t_nominal_value=1  phi_specify=on  phi_priority=High  phi=0 rad  phi_nominal_specify=off  phi_nominal_unit=rad  phi_nominal_value=1
      settings: SourceProductName=Foundation Library
  Inertia : fl_lib/Mechanical/Rotational Elements/Inertia  inertia=J kg*m^2  w_specify=off  w_priority=High  w=0 rad/s  w_nominal_specify=off  w_nominal_unit=rad/s  w_nominal_value=1  t_specify=off  t_priority=High  t=0 N*m  t_nominal_specify=off  t_nominal_unit=N*m  t_nominal_value=1
      settings: SourceProductName=Foundation Library
  LVDT Position Sensor System 10V/mm1 : Subsystem
  Mechanical Rotational Reference : fl_lib/Mechanical/Rotational Elements/Mechanical Rotational Reference
      settings: SourceProductName=Foundation Library
  Motor Control Circuit : Subsystem  Tag=PublishSubsystem
  Rotation : Subsystem
      mask Display: disp('A')
  Rotational Electromechanical Converter : fl_lib/Electrical/Electrical Elements/Rotational Electromechanical Converter  K=Kt V/(rad/s)  i_specify=off  i_priority=High  i=0 A  i_nominal_specify=off  i_nominal_unit=A  i_nominal_value=1  v_specify=off  v_priority=High  v=0 V  v_nominal_specify=off  v_nominal_unit=V  v_nominal_value=1  t_specify=off  t_priority=High  t=0 N*m  t_nominal_specify=off  t_nominal_unit=N*m  t_nominal_value=1  w_specify=off  w_priority=High  w=0 rad/s  w_nominal_specify=off  w_nominal_unit=rad/s  w_nominal_value=1
      settings: SourceProductName=Foundation Library
  Rotor Inductance : fl_lib/Electrical/Electrical Elements/Inductor  l=L H  r=0 Ohm  g=1e-09 1/Ohm  i_specify=off  i_priority=High  i=0 A  i_nominal_specify=off  i_nominal_unit=A  i_nominal_value=1  v_specify=off  v_priority=High  v=0 V  v_nominal_specify=off  v_nominal_unit=V  v_nominal_value=1  i_L_specify=on  i_L_priority=High  i_L=0 A  i_L_nominal_specify=off  i_L_nominal_unit=A  i_L_nominal_value=1
      settings: SourceProductName=Foundation Library
  Rotor Resistance : fl_lib/Electrical/Electrical Elements/Resistor  Tag=Factory Generic  R=R Ohm  i_specify=off  i_priority=High  i=0 A  i_nominal_specify=off  i_nominal_unit=A  i_nominal_value=1  v_specify=off  v_priority=High  v=0 V  v_nominal_specify=off  v_nominal_unit=V  v_nominal_value=1
      settings: SourceProductName=Foundation Library
  Vi : PMIOPort  Side=Left
  A : PMIOPort  Port=2  Side=Right
  connections:
  Damper/RConn1 -- Hard Stop/RConn1 -- Rotational Electromechanical Converter/RConn2 -- Mechanical Rotational Reference/LConn1
  Rotational Electromechanical Converter/LConn1 -- Rotor Inductance/RConn1
  Rotor Inductance/LConn1 -- Rotor Resistance/RConn1
  Motor Control Circuit/RConn1 -- Rotor Resistance/LConn1
  Vi/RConn1 -- Motor Control Circuit/LConn1
  LVDT Position Sensor System 10V/mm1/RConn2 -- Motor Control Circuit/LConn2
  Rotational Electromechanical Converter/RConn1 -- Motor Control Circuit/RConn2
  Electrical Reference1/LConn1 -- LVDT Position Sensor System 10V/mm1/RConn1
  A/RConn1 -- Rotation/RConn1 -- LVDT Position Sensor System 10V/mm1/LConn1
  Hard Stop/LConn1 -- Rotation/LConn1 -- Rotational Electromechanical Converter/LConn2 -- Inertia/LConn1 -- Damper/LConn1

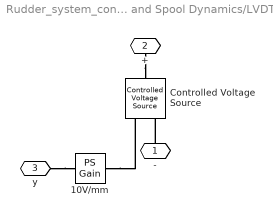
== system Rudder_system_control2020_3/Spool Valve/Torque Motor, Controller and Spool Dynamics/LVDT Position Sensor System 10V//mm1 ==
  10V/mm : fl_lib/Physical Signals/Functions/PS Gain  gain=10 V/mm
      settings: SourceProductName=Foundation Library
  Controlled Voltage Source : fl_lib/Electrical/Electrical Sources/Controlled Voltage Source
      settings: SourceProductName=Foundation Library
  - : PMIOPort  Side=Right
  + : PMIOPort  Port=2  Side=Right
  y : PMIOPort  Port=3  Side=Left
  connections:
  y/RConn1 -- 10V/mm/LConn1
  -/RConn1 -- Controlled Voltage Source/RConn2
  +/RConn1 -- Controlled Voltage Source/LConn1
  10V/mm/RConn1 -- Controlled Voltage Source/RConn1

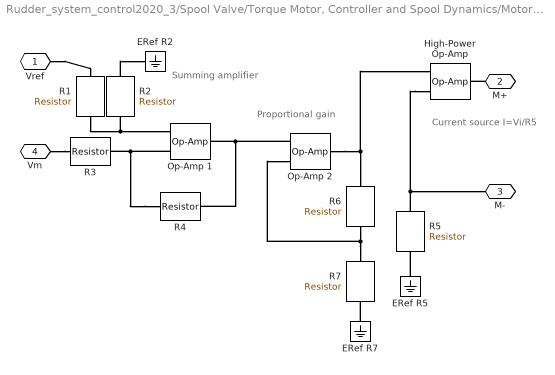
== system Rudder_system_control2020_3/Spool Valve/Torque Motor, Controller and Spool Dynamics/Motor Control Circuit ==
  note: Current source
      | I=Vi/R5
  note: Summing
      | amplifier
  note: Proportional gain
  ERef R2 : fl_lib/Electrical/Electrical Elements/Electrical Reference
      settings: SourceProductName=Foundation Library
  ERef R5 : fl_lib/Electrical/Electrical Elements/Electrical Reference
      settings: SourceProductName=Foundation Library
  ERef R7 : fl_lib/Electrical/Electrical Elements/Electrical Reference
      settings: SourceProductName=Foundation Library
  High-Power Op-Amp : fl_lib/Electrical/Electrical Elements/Op-Amp  outI_specify=off  outI_priority=High  outI=0 A  outI_nominal_specify=off  outI_nominal_unit=A  outI_nominal_value=1
      settings: SourceProductName=Foundation Library
  Op-Amp 1 : fl_lib/Electrical/Electrical Elements/Op-Amp  outI_specify=off  outI_priority=High  outI=0 A  outI_nominal_specify=off  outI_nominal_unit=A  outI_nominal_value=1
      settings: SourceProductName=Foundation Library
  Op-Amp 2 : fl_lib/Electrical/Electrical Elements/Op-Amp  outI_specify=off  outI_priority=High  outI=0 A  outI_nominal_specify=off  outI_nominal_unit=A  outI_nominal_value=1
      settings: SourceProductName=Foundation Library
  R1 : fl_lib/Electrical/Electrical Elements/Resistor  R=R_controller(1) Ohm  i_specify=off  i_priority=High  i=0 A  i_nominal_specify=off  i_nominal_unit=A  i_nominal_value=1  v_specify=off  v_priority=High  v=0 V  v_nominal_specify=off  v_nominal_unit=V  v_nominal_value=1
      settings: SourceProductName=Foundation Library
  R2 : fl_lib/Electrical/Electrical Elements/Resistor  R=R_controller(2) Ohm  i_specify=off  i_priority=High  i=0 A  i_nominal_specify=off  i_nominal_unit=A  i_nominal_value=1  v_specify=off  v_priority=High  v=0 V  v_nominal_specify=off  v_nominal_unit=V  v_nominal_value=1
      settings: SourceProductName=Foundation Library
  R3 : fl_lib/Electrical/Electrical Elements/Resistor  R=R_controller(3) Ohm  i_specify=off  i_priority=High  i=0 A  i_nominal_specify=off  i_nominal_unit=A  i_nominal_value=1  v_specify=off  v_priority=High  v=0 V  v_nominal_specify=off  v_nominal_unit=V  v_nominal_value=1
      settings: SourceProductName=Foundation Library
  R4 : fl_lib/Electrical/Electrical Elements/Resistor  R=R_controller(4) Ohm  i_specify=off  i_priority=High  i=0 A  i_nominal_specify=off  i_nominal_unit=A  i_nominal_value=1  v_specify=off  v_priority=High  v=0 V  v_nominal_specify=off  v_nominal_unit=V  v_nominal_value=1
      settings: SourceProductName=Foundation Library
  R5 : fl_lib/Electrical/Electrical Elements/Resistor  R=R_controller(5) Ohm  i_specify=off  i_priority=High  i=0 A  i_nominal_specify=off  i_nominal_unit=A  i_nominal_value=1  v_specify=off  v_priority=High  v=0 V  v_nominal_specify=off  v_nominal_unit=V  v_nominal_value=1
      settings: SourceProductName=Foundation Library
  R6 : fl_lib/Electrical/Electrical Elements/Resistor  R=R_controller(6) Ohm  i_specify=off  i_priority=High  i=0 A  i_nominal_specify=off  i_nominal_unit=A  i_nominal_value=1  v_specify=off  v_priority=High  v=0 V  v_nominal_specify=off  v_nominal_unit=V  v_nominal_value=1
      settings: SourceProductName=Foundation Library
  R7 : fl_lib/Electrical/Electrical Elements/Resistor  R=R_controller(7) Ohm  i_specify=off  i_priority=High  i=0 A  i_nominal_specify=off  i_nominal_unit=A  i_nominal_value=1  v_specify=off  v_priority=High  v=0 V  v_nominal_specify=off  v_nominal_unit=V  v_nominal_value=1
      settings: SourceProductName=Foundation Library
  Vref : PMIOPort  Side=Left
  M+ : PMIOPort  Port=2  Side=Right
  M- : PMIOPort  Port=3  Side=Right
  Vm : PMIOPort  Port=4  Side=Left
  connections:
  ERef R7/LConn1 -- R7/RConn1
  R2/RConn1 -- ERef R2/LConn1
  ERef R5/LConn1 -- R5/RConn1
  Op-Amp 2/RConn1 -- High-Power Op-Amp/LConn1 -- R6/LConn1
  High-Power Op-Amp/LConn2 -- M-/RConn1 -- R5/LConn1
  R2/LConn1 -- Op-Amp 1/LConn1 -- R1/RConn1
  R4/LConn1 -- Op-Amp 1/LConn2 -- R3/RConn1
  Op-Amp 2/LConn1 -- Op-Amp 1/RConn1 -- R4/RConn1
  R7/LConn1 -- Op-Amp 2/LConn2 -- R6/RConn1
  Vref/RConn1 -- R1/LConn1
  M+/RConn1 -- High-Power Op-Amp/RConn1
  Vm/RConn1 -- R3/LConn1

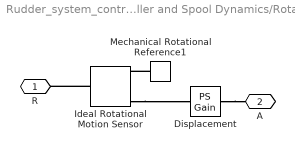
== system Rudder_system_control2020_3/Spool Valve/Torque Motor, Controller and Spool Dynamics/Rotation ==
  Displacement : fl_lib/Physical Signals/Functions/PS Gain  gain=G m/rad
      settings: SourceProductName=Foundation Library
  Ideal Rotational Motion Sensor : fl_lib/Mechanical/Mechanical Sensors/Ideal Rotational Motion Sensor  wrap_angle=simscape.enum.onoff.off  offset=0 rad
      settings: SourceProductName=Foundation Library
  Mechanical Rotational Reference1 : fl_lib/Mechanical/Rotational Elements/Mechanical Rotational Reference
      settings: SourceProductName=Foundation Library
  R : PMIOPort  Side=Left
  A : PMIOPort  Port=2  Side=Right
  connections:
  Mechanical Rotational Reference1/LConn1 -- Ideal Rotational Motion Sensor/RConn1
  Ideal Rotational Motion Sensor/RConn3 -- Displacement/LConn1
  Displacement/RConn1 -- A/RConn1
  Ideal Rotational Motion Sensor/LConn1 -- R/RConn1
